simulink model "complete_model_sim"  (R2023b)
settings: Solver=VariableStepAuto  StartTime=0.0  StopTime=5e3  RelTol=1e-3
values from neighbouring files (symbols this model uses):
  a = 6.851221970532768e+03    (= 6851.22197053)    [complete_model.m]
  alpha1 = 0.05    [complete_model.m]
  alpha2 = 0.15    [complete_model.m]
  alpha3 = 0.8    [complete_model.m]
  D = squeeze(out.D)    [complete_model.m]
  e = 0.001830122216180    (= 0.00183012221618)    [complete_model.m]
  FOV_earth = deg2rad(33)    [complete_model.m]
  freq_earth = 30    [complete_model.m]
  freq_mag = 30    [complete_model.m]
  freq_sun = 30    [complete_model.m]
  H0 = sqrt(g01^2+g11^2+h11^2)*1e-9    [complete_model.m]
  I = I + (y(i + 1) + y(i) ) * (t(i + 1) - t(i)) * 0.5    [compute_integral.m]
  incl = deg2rad(11.5)    [complete_model.m]
  jb = [0.01; 0.05; 0.01]    [complete_model.m]
  k_gain = (4*pi/T) * (1 + sin(chsi)) * I1_retr    [complete_model.m]
  mu = astroConstants(13)    [complete_model.m]
  n = sqrt(mu/a^3)    [complete_model.m]
  omega0 = -0.06 + 0.12 * rand(3,1)    [complete_model.m]
  omegaE = deg2rad(15)/3600    [complete_model.m]
  rs = -rr    [complete_model.m]
  Rt = astroConstants(23)    [complete_model.m]
  s0 = 2*pi*rand(3,1)    [complete_model.m]
  tol = 0.2    [complete_model.m]
undefined symbols (not defined in the file or in its folder): FOV_sun, Iinv, magnitude
libraries: simulink x16, vrlib x13, matrix_library x12, cstblocks x6, dspsolvers x4, sharedutil x2, aerolibutil x2, dspfactors x1, dspmathops x1
(part 1 of 2)
settings Model: Creator=marcellopareschi  LastModifiedBy=turcu

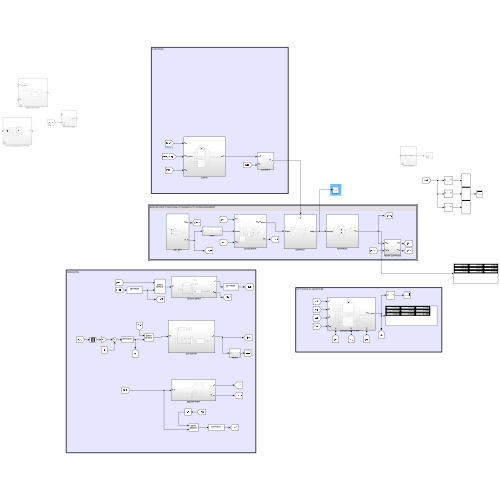
[thumbnail: Simulink's stored preview of the top-level diagram]
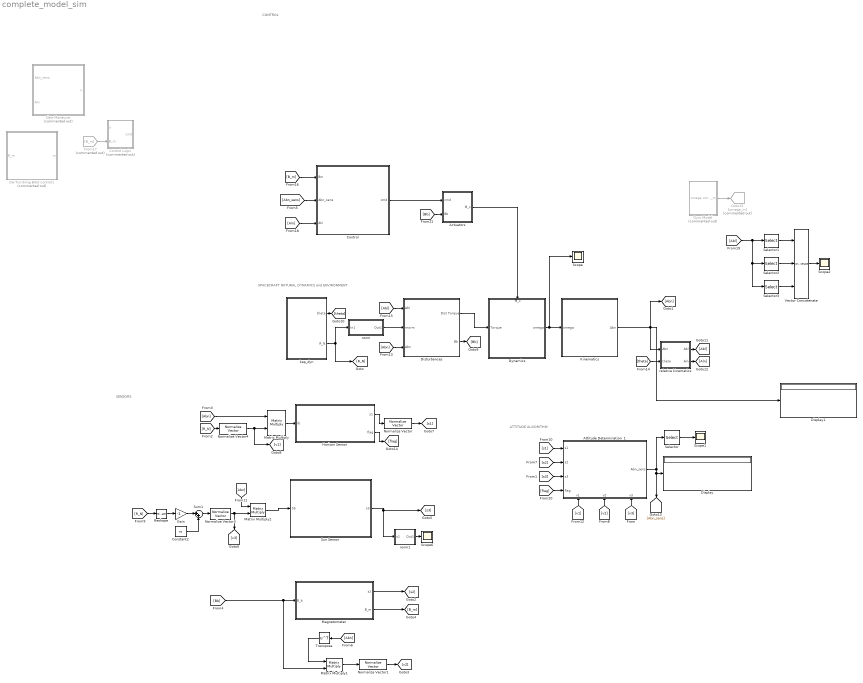
== system complete_model_sim ==
  note: SPACECRAFT NATURAL DYNAMICS and ENVIRONMENT
  note: CONTROL
  note: ATTITUDE ALGORITHM
  note: SENSORS
  " Actuators" : Subsystem
  Attitude Determination  1 : Subsystem
      settings: PortSchema="{\"entries\":[{\"content\":{\"sides\":[{\"content\":{\"connectorIds\":[\"In1\",\"In2\",\"In3\",\"In4\"]},\"type\":\"ConnectorPlacement.EquallySpacedRectSide\",\"uuid\":\"730966cf-d0d7-44a0-92f0-b5324480e7cc\"},{\"content\":{\"connectorIds\":[\"Out1\"],\"side\":\"RIGHT\"},\"type\":\"ConnectorPlacement.EquallySpacedRectSide\",\"uuid\":\"c83e6b57-46fe-4a45-9824-d3495e15bf6a\"},{\"content\":{\"side\":\"TOP\"},\"type\":\"ConnectorPlacement.EquallySpacedRectSide\",\"uuid\":\"4938c298-c2b3-45b7-bcb0-70b8132dabc6\"},{\"content\":{\"connectorIds\":[\"In5\",\"In6\",\"In7\"],\"side\":\"BOTTOM\"},\"type\":\"ConnectorPlacement.EquallySpacedRectSide\",\"uuid\":\"6d6a244e-80db-423b-a0a5-9a5face48fcb\"}]},\"type\":\"ConnectorPlacement.EquallySpacedConnector\",\"uuid\":\"7eb6767d-3ff0-4577-86c9-ebc5e763f220\"}],\"packageUris\":[\"http://schema.mathworks.com/mf0/Connector/R2020b\"],\"version\":\"1.0\"}"
  Constant2 : Constant  Value=rs
  Control : Subsystem
  Control Logic : Subsystem  Commented=on
  De-Tumbling Bdot control1 : Subsystem  Commented=on
  Display : Display
  Display1 : Display
  Disturbances : Subsystem
  Dynamics : Subsystem
      settings: PortSchema="{\"entries\":[{\"content\":{\"sides\":[{\"content\":{\"connectorIds\":[\"In1\"]},\"type\":\"ConnectorPlacement.EquallySpacedRectSide\",\"uuid\":\"c50eaaef-bc5a-4b30-975a-dad3b72c53e1\"},{\"content\":{\"connectorIds\":[\"Out1\"],\"side\":\"RIGHT\"},\"type\":\"ConnectorPlacement.EquallySpacedRectSide\",\"uuid\":\"08d23e91-5daf-4f03-95f9-71d6696597c3\"},{\"content\":{\"connectorIds\":[\"In2\"],\"side\":\"TOP\"},\"type\":\"ConnectorPlacement.EquallySpacedRectSide\",\"uuid\":\"7ec65280-cc3e-44b1-8843-81c3a216d755\"}]},\"type\":\"ConnectorPlacement.EquallySpacedConnector\",\"uuid\":\"721d018a-ab6c-4a15-8dbf-409a72b03ba1\"}],\"packageUris\":[\"http://schema.mathworks.com/mf0/Connector/R2020b\"],\"version\":\"1.0\"}"
  From17 : From  Commented=on  GotoTag=B_m
  Gain : Gain  Gain=-1
  Goto15 : Goto  Commented=on  GotoTag=omega_m
  Gyro Model : Subsystem  Commented=on
  Horizon Sensor : Subsystem
  Kinematics : Subsystem
  Magnetometer : Subsystem
  Matrix Multiply : Product  Multiplication=Matrix(*)
  Matrix Multiply1 : Product  Multiplication=Matrix(*)
  Matrix Multiply2 : Product  Multiplication=Matrix(*)
  Normalize Vector{,1,3..4} (4 alike) : vrlib/Utilities/Normalize Vector  maxzero=0
  Reshape : Reshape  OutputDimensionality=Column vector (2-D)
  Scope{,1..2,6} (4 alike) : Scope
  Selector : Selector  NumberOfDimensions=2  InputPortWidth=3  IndexOptions=Index vector (dialog),Index vector (dialog)  Indices=1,1  OutputSizes=1,1
  Selector1 : Selector  NumberOfDimensions=2  InputPortWidth=3  IndexOptions=Index vector (dialog),Index vector (dialog)  Indices=3,2  OutputSizes=1,1
  Selector2 : Selector  NumberOfDimensions=2  InputPortWidth=3  IndexOptions=Index vector (dialog),Index vector (dialog)  Indices=1,3  OutputSizes=1,1
  Selector3 : Selector  NumberOfDimensions=2  InputPortWidth=3  IndexOptions=Index vector (dialog),Index vector (dialog)  Indices=2,1  OutputSizes=1,1
  Slew Maneuver : Subsystem  Commented=on
  Sum1 : Sum  Inputs=|++
  Sun Sensor : Subsystem
  Transpose : Math  Operator=transpose
  Vector Concatenate : Concatenate  NumInputs=3
  kep_dyn : Subsystem
  norm : Subsystem
  norm1 : Subsystem
  relative kinematics : Subsystem
  wires:
  Normalize Vector3/1 -> Matrix Multiply2/2, [v3]
  Magnetometer/1(s2) -> [s2]
  Disturbances/2(Bb) -> [Bb]
  [Abn] -> Transpose/1
  Matrix Multiply1/1 -> Normalize Vector1/1
  Transpose/1 -> Matrix Multiply1/1
  [theta] -> relative kinematics/2(theta)
  [v1] -> Attitude Determination  1/5(v1)
  [Abn] -> Matrix Multiply/1
  [R_N] -> Reshape/1
  Gain/1 -> Sum1/1
  [Bb] -> Matrix Multiply1/2, Magnetometer/1(B_b)
  Normalize Vector4/1 -> [v1], Matrix Multiply/2
  [s3] -> Attitude Determination  1/3(s3)
  Normalize Vector1/1 -> [v2]
  " Actuators"/1(M_c) -> Dynamics/2(M_c)
  Magnetometer/2("B_m ") -> [B_m]
  Sun Sensor/1(s3) -> norm1/1(s1), [s3]
  [R_N] -> Normalize Vector4/1
  Constant2/1 -> Sum1/2
  kep_dyn/1(theta) -> [theta]
  [s2] -> Attitude Determination  1/2(s2)
  Matrix Multiply/1 -> Horizon Sensor/1(rb)
  Reshape/1 -> Gain/1
  [Abl] -> Disturbances/1(Abl)
  Normalize Vector/1 -> [s1]
  [v3] -> Attitude Determination  1/7(v3)
  [s1] -> Attitude Determination  1/1(s1)
  kep_dyn/2(R_N) -> [R_N], norm/1(In1)
  Sum1/1 -> Normalize Vector3/1
  Attitude Determination  1/1(Abn_sens) -> [Abn_sens], Display/1, Selector/1
  relative kinematics/1(Abl) -> [Abl]
  Kinematics/1(Abn) -> [Abn], Display1/1, relative kinematics/1(Abn)
  relative kinematics/2(Aln) -> [Aln]
  Selector/1 -> Scope1/1
  [Abn] -> Disturbances/3(Abn)
  norm/1(Out1) -> Disturbances/2(rnorm)
  [Abn] -> Matrix Multiply2/1
  Disturbances/1(Dist Torque) -> Dynamics/1(Torque)
  Dynamics/1(omega) -> Scope/1, Kinematics/1(omega)
  [v2] -> Attitude Determination  1/6(v2)
  Horizon Sensor/1(s1) -> Normalize Vector/1
  Matrix Multiply2/1 -> Sun Sensor/1(Sb)
  norm1/1(Out1) -> Scope6/1
  Gyro Model/1(omega_m) -> Goto15/1
  [Bb] -> " Actuators"/2(Bb)
  From17/1 -> Control Logic/2(B_m)
  [B_m] -> Control/1(Bm)
  [Abn_sens] -> Control/2(Abn_sens)
  [Aln] -> Control/3(Aln)
  Control/1(cmd) -> " Actuators"/1(cmd)
  [Abl] -> Selector3/1, Selector2/1, Selector1/1
  Selector2/1 -> Vector Concatenate/2
  Selector3/1 -> Vector Concatenate/3
  Selector1/1 -> Vector Concatenate/1
  Vector Concatenate/1 -> Scope2/1
  Horizon Sensor/2(flag) -> [flag]
  [flag] -> Attitude Determination  1/4(flag)

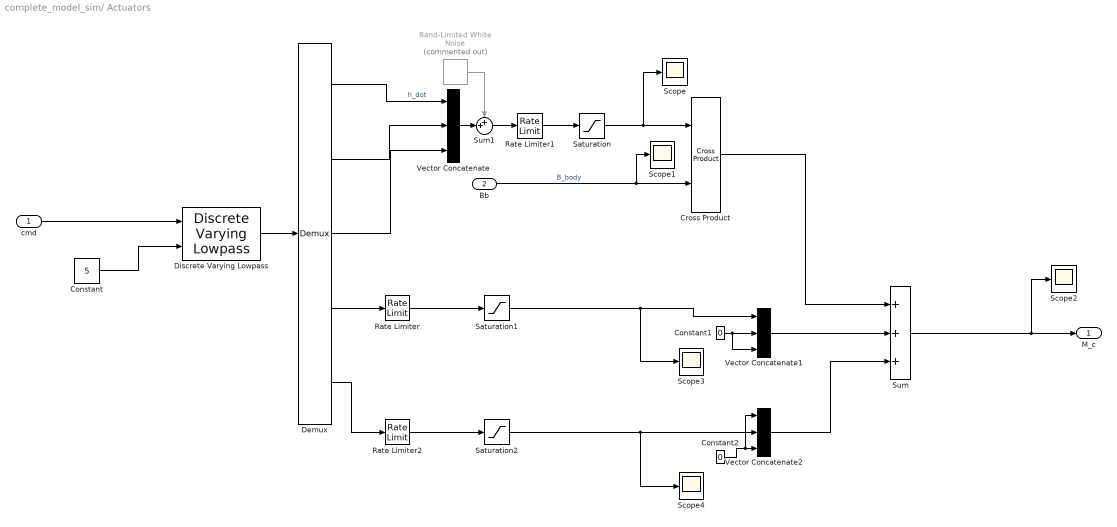
== system complete_model_sim/ Actuators ==
  cmd : Inport
  Bb : Inport  Port=2
  Band-Limited White Noise : simulink/Sources/Band-Limited White Noise  Commented=on  Cov=[0.1]  Ts=1/30  seed=[23341]
  Constant : Constant  Value=5
  Constant1 : Constant  Value=0
  Constant2 : Constant  Value=0
  Cross Product : matrix_library/Cross Product
  Demux : Demux  Outputs=5
  Discrete Varying Lowpass : cstblocks/Linear Parameter Varying/Discrete Varying Lowpass  N=2  w0=0  Ts=1/30
  Rate Limiter : RateLimiter
  Rate Limiter1 : RateLimiter  RisingSlewLimit=10  FallingSlewLimit=-10
  Rate Limiter2 : RateLimiter
  Saturation : Saturate  UpperLimit=150  LowerLimit=-150
  Saturation1 : Saturate
  Saturation2 : Saturate
  Scope{,1..4} (5 alike) : Scope
  Sum : Sum  Inputs=+++
  Sum1 : Sum  Inputs=++|
  Vector Concatenate : Concatenate  NumInputs=3
  Vector Concatenate1 : Concatenate  NumInputs=3
  Vector Concatenate2 : Concatenate  NumInputs=3
  M_c : Outport
  wires:
  Bb/1 -> Scope1/1, Cross Product/2  "B_body"
  Rate Limiter1/1 -> Saturation/1
  Band-Limited White Noise/1 -> Sum1/1
  Sum1/1 -> Rate Limiter1/1
  Saturation/1 -> Scope/1, Cross Product/1
  Vector Concatenate/1 -> Sum1/2
  Constant1/1 -> Vector Concatenate1/3, Vector Concatenate1/2
  Sum/1 -> Scope2/1, M_c/1
  Rate Limiter/1 -> Saturation1/1
  Saturation1/1 -> Scope3/1, Vector Concatenate1/1
  Demux/1 -> Vector Concatenate/1  "h_dot"
  Demux/2 -> Vector Concatenate/2
  Demux/3 -> Vector Concatenate/3
  Demux/4 -> Rate Limiter/1
  Saturation2/1 -> Vector Concatenate2/2, Scope4/1
  Constant2/1 -> Vector Concatenate2/1, Vector Concatenate2/3
  Rate Limiter2/1 -> Saturation2/1
  Demux/5 -> Rate Limiter2/1
  Vector Concatenate1/1 -> Sum/2
  Cross Product/1 -> Sum/1
  Vector Concatenate2/1 -> Sum/3
  Constant/1 -> Discrete Varying Lowpass/2
  Discrete Varying Lowpass/1 -> Demux/1
  cmd/1 -> Discrete Varying Lowpass/1

== system complete_model_sim/Attitude Determination  1 ==
  s1 : Inport
  s2 : Inport  Port=2
  s3 : Inport  Port=3
  flag : Inport  Port=4
  v1 : Inport  Port=5
  v2 : Inport  Port=6
  v3 : Inport  Port=7
  Enabled Subsystem : Subsystem  TreatAsAtomicUnit=on
  Merge : Merge
  NOT : Logic  Operator=NOT  IconShape=distinctive  AllPortsSameDT=off  OutDataTypeStr=boolean
  Statistical Method : Subsystem  TreatAsAtomicUnit=on
  Abn_sens : Outport
  wires:
  flag/1 -> NOT/1, Statistical Method/Enable
  s1/1 -> Statistical Method/1(s1)
  s2/1 -> Enabled Subsystem/1(q), Statistical Method/2(s2)
  s3/1 -> Enabled Subsystem/2(p), Statistical Method/3(s3)
  v1/1 -> Statistical Method/4(v1)
  v2/1 -> Enabled Subsystem/3(b), Statistical Method/5(v2)
  v3/1 -> Enabled Subsystem/4(a), Statistical Method/6(v3)
  NOT/1 -> Enabled Subsystem/Enable
  Statistical Method/1(Abn_sens) -> Merge/1
  Enabled Subsystem/1(A_bn_sens) -> Merge/2
  Merge/1 -> Abn_sens/1

== system complete_model_sim/Control ==
  Bm : Inport
  Abn_sens : Inport  Port=2
  Aln : Inport  Port=3
  De-Tumbling Bdot control1 : Subsystem
  Merge : Merge
  NOT : Logic  Operator=NOT  IconShape=distinctive  AllPortsSameDT=off  OutDataTypeStr=boolean
  Scope1 : Scope
  Slew Maneuver : Subsystem
  Unit Delay : UnitDelay  InitialCondition=1  SampleTime=-1  HasFrameUpgradeWarning=on
  cmd : Outport
  wires:
  Unit Delay/1 -> NOT/1, Scope1/1, De-Tumbling Bdot control1/Enable
  De-Tumbling Bdot control1/2(flag) -> Unit Delay/1
  Bm/1 -> Slew Maneuver/3(B_m), De-Tumbling Bdot control1/1(B_m)
  Abn_sens/1 -> Slew Maneuver/1(Abn_sens)
  Aln/1 -> Slew Maneuver/2(Aln)
  NOT/1 -> Slew Maneuver/Enable
  Slew Maneuver/1(cmd) -> Merge/2
  De-Tumbling Bdot control1/1(cmd) -> Merge/1
  Merge/1 -> cmd/1

== system complete_model_sim/Control Logic ==
  u : Inport
  B_m : Inport  Port=2
  Abs1 : Abs  SaturateOnIntegerOverflow=off
  Compare To Constant : simulink/Logic and Bit Operations/Compare To Constant  relop=>  const=1e-5  OutDataTypeStr=boolean
  Discrete Derivative : simulink/Discrete/Discrete Derivative  gainval=1.0  ICPrevScaledInput=0.0  OutMin=[]  OutMax=[]  OutDataType=fixdt(1, 16)  OutScaling=2^-10  DoSatur=off
  Merge1 : Merge
  NOT : Logic  Operator=NOT  IconShape=distinctive  AllPortsSameDT=off  OutDataTypeStr=boolean
  Scope : Scope
  Selector1 : Selector  InputPortWidth=3  IndexOptions=Index vector (dialog)  Indices=1  OutputSizes=1
  Subsystem : Subsystem
  Subsystem1 : Subsystem
  norm : Subsystem
  cmd : Outport
  wires:
  Abs1/1 -> Compare To Constant/1
  Selector1/1 -> Abs1/1
  NOT/1 -> Subsystem/Enable
  Subsystem1/1(Out1) -> Merge1/1
  Compare To Constant/1 -> NOT/1, Subsystem1/Enable
  Subsystem/1(Out1) -> Merge1/2
  B_m/1 -> Discrete Derivative/1, Selector1/1, Subsystem/1(Bm), Subsystem1/1(B_m)
  u/1 -> Subsystem/2(u), Subsystem1/2(u)
  Merge1/1 -> cmd/1
  Discrete Derivative/1 -> norm/1(In1)
  norm/1(Out1) -> Scope/1

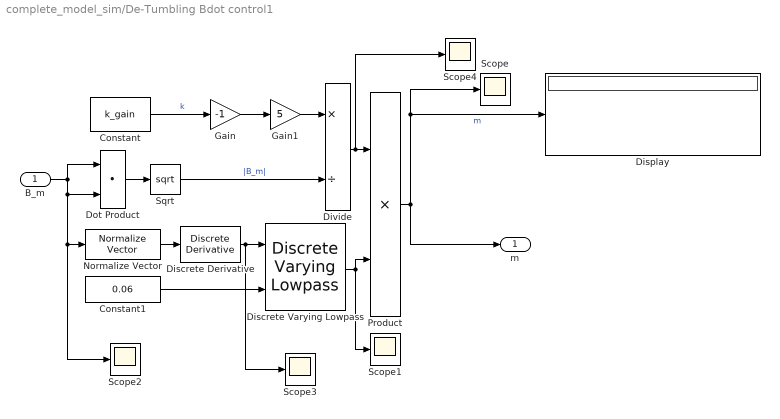
== system complete_model_sim/De-Tumbling Bdot control1 ==
  B_m : Inport
  Constant : Constant  Value=k_gain
  Constant1 : Constant  Value=0.06  SampleTime=1/30
  Discrete Derivative : simulink/Discrete/Discrete Derivative  gainval=1.0  ICPrevScaledInput=0.0  OutMin=[]  OutMax=[]  OutDataType=fixdt(1, 16)  OutScaling=2^-10  DoSatur=off
  Discrete Varying Lowpass : cstblocks/Linear Parameter Varying/Discrete Varying Lowpass  N=1  w0=0  Ts=1/30
  Display : Display
  Divide : Product  Inputs=*/
  Dot Product : DotProduct  OutDataTypeStr=Inherit: Inherit via internal rule
  Gain : Gain  Gain=-1
  Gain1 : Gain  Gain=5
  Normalize Vector : vrlib/Utilities/Normalize Vector  maxzero=0
  Product : Product
  Scope{,1..4} (5 alike) : Scope
  Sqrt : Sqrt
  m : Outport
  wires:
  Dot Product/1 -> Sqrt/1
  Constant/1 -> Gain/1  "k"
  Gain/1 -> Gain1/1
  Divide/1 -> Scope4/1, Product/1
  Product/1 -> m/1, Scope/1, Display/1  "m"
  Sqrt/1 -> Divide/2  "|B_m|"
  Gain1/1 -> Divide/1
  Normalize Vector/1 -> Discrete Derivative/1
  B_m/1 -> Dot Product/2, Scope2/1, Normalize Vector/1, Dot Product/1
  Discrete Derivative/1 -> Scope3/1, Discrete Varying Lowpass/1
  Discrete Varying Lowpass/1 -> Scope1/1, Product/2
  Constant1/1 -> Discrete Varying Lowpass/2

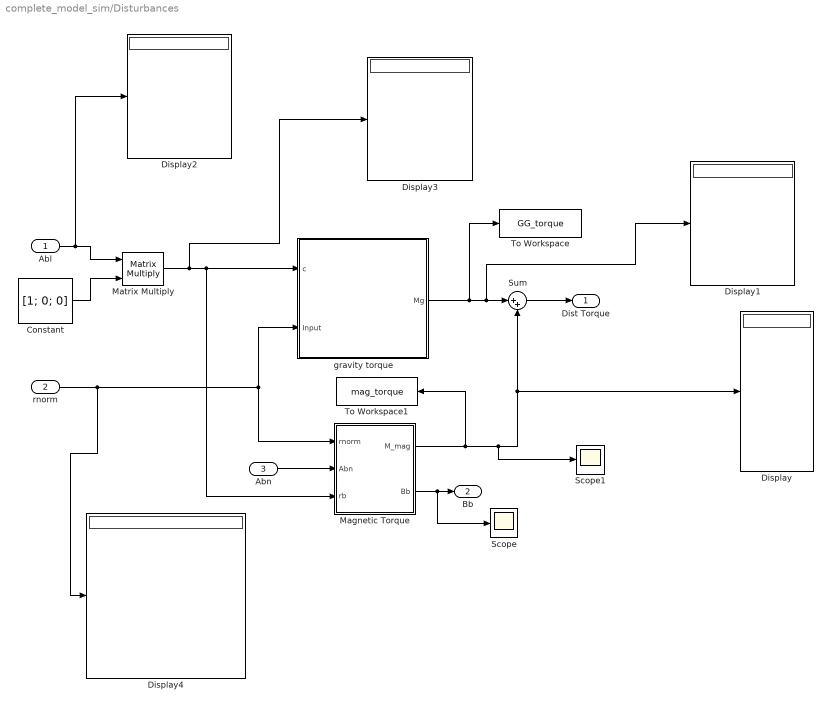
== system complete_model_sim/Disturbances ==
  Abl : Inport
  rnorm : Inport  Port=2
  Abn : Inport  Port=3
  Constant : Constant  Value=[1; 0; 0]
  Display{,1..4} (5 alike) : Display
  "Magnetic Torque " : Subsystem
  Matrix Multiply : Product  Multiplication=Matrix(*)
  Scope : Scope
  Scope1 : Scope
  Sum : Sum  Inputs=|++
  To Workspace : ToWorkspace  VariableName=GG_torque  SampleTime=-1
  To Workspace1 : ToWorkspace  VariableName=mag_torque  SampleTime=-1
  gravity torque : Subsystem
  Dist Torque : Outport
  Bb : Outport  Port=2
  wires:
  Abl/1 -> Display2/1, Matrix Multiply/1
  Constant/1 -> Matrix Multiply/2
  Matrix Multiply/1 -> Display3/1, "Magnetic Torque "/3(rb), gravity torque/1(c)
  rnorm/1 -> Display4/1, "Magnetic Torque "/1(rnorm), gravity torque/2(Input)
  Abn/1 -> "Magnetic Torque "/2(Abn)
  gravity torque/1(Mg) -> To Workspace/1, Display1/1, Sum/1
  "Magnetic Torque "/1(M_mag) -> To Workspace1/1, Scope1/1, Sum/2, Display/1
  Sum/1 -> Dist Torque/1
  "Magnetic Torque "/2(Bb) -> Scope/1, Bb/1

== system complete_model_sim/Dynamics ==
  Torque : Inport
  M_c : Inport  Port=2
  Constant : Constant  Value=I
  Constant1 : Constant  Value=Iinv
  Cross Product : matrix_library/Cross Product
  Integrator : Integrator  InitialCondition=omega0
  Product : Product  Multiplication=Matrix(*)
  Product1 : Product  Multiplication=Matrix(*)
  Scope : Scope
  Scope1 : Scope
  Sum : Sum  Inputs=+++
  To Workspace : ToWorkspace  VariableName=omegab  SampleTime=-1
  omega : Outport
  wires:
  Constant/1 -> Product/1
  Product1/1 -> Integrator/1
  Integrator/1 -> Product/2, Cross Product/2, Scope/1, To Workspace/1, omega/1
  Product/1 -> Cross Product/1
  Constant1/1 -> Product1/1
  Cross Product/1 -> Sum/2
  Sum/1 -> Product1/2
  Torque/1 -> Sum/3
  M_c/1 -> Scope1/1, Sum/1

== system complete_model_sim/Gyro Model ==
  omega : Inport
  Constant : Constant
  Discrete Varying Lowpass : cstblocks/Linear Parameter Varying/Discrete Varying Lowpass  N=2  w0=0  Ts=1
  Integrator : Integrator
  Random Number : RandomNumber  Variance=(9.6963*1e-7)^2  SampleTime=0.1
  Random Number1 : RandomNumber  Variance=(9.6963*1e-7)^2  SampleTime=0.1
  Random Number2 : RandomNumber  Variance=(9.6963*1e-7)^2  SampleTime=0.1
  Random Number3 : RandomNumber  Variance=(2.3522*1e-5)^2  SampleTime=0.1
  Random Number4 : RandomNumber  Variance=(2.3522*1e-5)^2  SampleTime=0.1
  Random Number5 : RandomNumber  Variance=(2.3522*1e-5)^2  SampleTime=0.1
  Sum : Sum  Inputs=+++
  Vector Concatenate : Concatenate  NumInputs=3
  Vector Concatenate1 : Concatenate  NumInputs=3
  omega_m : Outport
  wires:
  Random Number1/1 -> Vector Concatenate/2
  Random Number/1 -> Vector Concatenate/1
  Random Number2/1 -> Vector Concatenate/3
  Vector Concatenate/1 -> Integrator/1
  Random Number3/1 -> Vector Concatenate1/1
  Random Number4/1 -> Vector Concatenate1/2
  Random Number5/1 -> Vector Concatenate1/3
  omega/1 -> Sum/2
  Vector Concatenate1/1 -> Sum/1
  Integrator/1 -> Sum/3
  Sum/1 -> Discrete Varying Lowpass/1
  Discrete Varying Lowpass/1 -> omega_m/1
  Constant/1 -> Discrete Varying Lowpass/2

== system complete_model_sim/Horizon Sensor ==
  rb : Inport
  EH sensor modeling : Subsystem
  FOV CHECK : Subsystem
  Product1 : Product
  Scope : Scope
  s1 : Outport
  flag : Outport  Port=2
  wires:
  rb/1 -> FOV CHECK/1(rb), Product1/2
  Product1/1 -> EH sensor modeling/1(rb)
  EH sensor modeling/1(q) -> s1/1  "direction of earth"
  FOV CHECK/1(b) -> Product1/1, Scope/1, flag/1

== system complete_model_sim/Kinematics ==
  omega : Inport
  Kinematics 312 : Subsystem
  Kinematics 313 : Subsystem
  Merge : Merge
  NOT : Logic  Operator=NOT  IconShape=distinctive  AllPortsSameDT=off  OutDataTypeStr=boolean
  System switcher : Subsystem
  To Workspace : ToWorkspace  VariableName=A  SaveFormat=Timeseries  SampleTime=-1
  Abn : Outport
  wires:
  NOT/1 -> Kinematics 313/Enable
  omega/1 -> Kinematics 312/1(w), Kinematics 313/1(w)
  System switcher/1(flag) -> Kinematics 312/Enable, NOT/1
  Kinematics 313/1(A) -> Merge/2
  Merge/1 -> Abn/1, To Workspace/1  "A"
  Kinematics 312/1(A) -> Merge/1

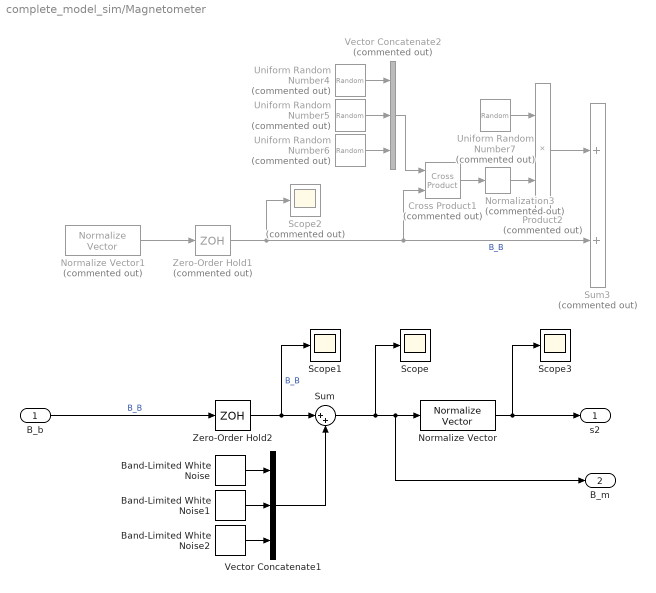
== system complete_model_sim/Magnetometer ==
  B_b : Inport
  Band-Limited White Noise : simulink/Sources/Band-Limited White Noise  Cov=[1.18^2 *1e-18]  Ts=1/30  seed=[23341]
  Band-Limited White Noise1 : simulink/Sources/Band-Limited White Noise  Cov=[1.18^2 *1e-18]  Ts=1/30  seed=[23341]
  Band-Limited White Noise2 : simulink/Sources/Band-Limited White Noise  Cov=[1.18^2 *1e-18]  Ts=1/30  seed=[23341]
  Cross Product1 : matrix_library/Cross Product  Commented=on
  Normalization3 : dspmathops/Normalization  Commented=on  NormType=2-norm  Bias=1e-10  NormOver=Each column  Dimension=1  roundingMode=Floor  overflowMode=off  accumDataTypeStr=Inherit: Same as product output  accumLastDataTypeStr=Inherit: Same as product output  outputDataTypeStr=Inherit: Same as product output  outputMin=[]  outputMax=[]  outputLastDataTypeStr=Inherit: Same as product output
  Normalize Vector : vrlib/Utilities/Normalize Vector  maxzero=0
  Normalize Vector1 : vrlib/Utilities/Normalize Vector  Commented=on  maxzero=0
  Product2 : Product  Commented=on
  Scope : Scope
  Scope1 : Scope
  Scope2 : Scope  Commented=on
  Scope3 : Scope
  Sum : Sum  Inputs=|++
  Sum3 : Sum  Commented=on
  Uniform Random Number4 : UniformRandomNumber  Commented=on  SampleTime=1/30
  Uniform Random Number5 : UniformRandomNumber  Commented=on  SampleTime=1/30
  Uniform Random Number6 : UniformRandomNumber  Commented=on  SampleTime=1/30
  Uniform Random Number7 : UniformRandomNumber  Commented=on  Minimum=0  Maximum=tan(deg2rad(0.5))*0.1  SampleTime=1/30
  Vector Concatenate1 : Concatenate  NumInputs=3
  Vector Concatenate2 : Concatenate  Commented=on  NumInputs=3
  Zero-Order Hold1 : ZeroOrderHold  Commented=on  SampleTime=1/30
  Zero-Order Hold2 : ZeroOrderHold  SampleTime=1/freq_mag
  s2 : Outport
  "B_m " : Outport  Port=2
  wires:
  Zero-Order Hold1/1 -> Cross Product1/2, Sum3/2, Scope2/1  "B_B"
  Product2/1 -> Sum3/1
  Normalization3/1 -> Product2/2
  Uniform Random Number4/1 -> Vector Concatenate2/1
  Uniform Random Number6/1 -> Vector Concatenate2/3
  Vector Concatenate2/1 -> Cross Product1/1
  Cross Product1/1 -> Normalization3/1
  Uniform Random Number5/1 -> Vector Concatenate2/2
  Uniform Random Number7/1 -> Product2/1
  Zero-Order Hold2/1 -> Scope1/1, Sum/1  "B_B"
  Band-Limited White Noise2/1 -> Vector Concatenate1/3
  Band-Limited White Noise1/1 -> Vector Concatenate1/2
  Band-Limited White Noise/1 -> Vector Concatenate1/1
  Normalize Vector/1 -> s2/1, Scope3/1
  Vector Concatenate1/1 -> Sum/2
  Sum/1 -> Scope/1, "B_m "/1, Normalize Vector/1
  Normalize Vector1/1 -> Zero-Order Hold1/1
  B_b/1 -> Zero-Order Hold2/1  "B_B"

== system complete_model_sim/Slew Maneuver ==
  Abn_sens : Inport
  Aln : Inport  Port=2
  Gain : Gain  Gain=-1
  Gain2 : Gain  Gain=-0.01
  Matrix Multiply : Product  Multiplication=Matrix(*)
  Scope : Scope
  Sum : Sum
  Transpose : Math  Operator=transpose
  compute alphadots : Subsystem
  compute alphas : Subsystem
  u : Outport
  wires:
  Aln/1 -> Transpose/1
  Transpose/1 -> Matrix Multiply/2
  Abn_sens/1 -> Matrix Multiply/1, compute alphadots/1(Abn)
  Matrix Multiply/1 -> compute alphas/1(Abl), compute alphadots/2(Abl)
  compute alphadots/1(Alphadots) -> Gain/1
  compute alphas/1(estimated state) -> Scope/1, Gain2/1
  Gain/1 -> Sum/1
  Gain2/1 -> Sum/2
  Sum/1 -> u/1

== system complete_model_sim/Sun Sensor ==
  Sb : Inport
  Constant : Constant
  FOV CHECK : Subsystem
  Product : Product
  Scope : Scope
  Sun Sensor Modeling : Subsystem
  s3 : Outport
  wires:
  Sb/1 -> Product/2, FOV CHECK/1(In1)  "Sb"
  Sun Sensor Modeling/1(s3) -> s3/1
  Product/1 -> Sun Sensor Modeling/1(Sb)  "Sb"
  Constant/1 -> Product/1
  FOV CHECK/1(b) -> Scope/1

== system complete_model_sim/kep_dyn ==
  A_np : Constant  Value=A_pn'
  Constant : Constant  Value=0
  Constant1 : Constant  Value=e
  Cos : Trigonometry  Operator=cos
  Integrator : Integrator
  Matrix Multiply : Product  Multiplication=Matrix(*)
  Product2 : Product
  Sin : Trigonometry
  Vector Concatenate : Concatenate  NumInputs=3
  r_norm : Subsystem
  theta integration : Subsystem
      settings: PortSchema="{\"entries\":[{\"content\":{\"sides\":[{\"content\":{\"connectorIds\":[\"In1\"]},\"type\":\"ConnectorPlacement.EquallySpacedRectSide\",\"uuid\":\"3f1b1ec9-07ed-4eb1-9e41-630dc5613e97\"},{\"content\":{\"connectorIds\":[\"Out1\",\"In2\"],\"side\":\"RIGHT\"},\"type\":\"ConnectorPlacement.EquallySpacedRectSide\",\"uuid\":\"22d0f7bc-714c-4365-a26c-07047ff4be14\"},{\"content\":{\"side\":\"TOP\"},\"type\":\"ConnectorPlacement.EquallySpacedRectSide\",\"uuid\":\"875f7006-d698-4730-93ae-1a7d05f24054\"}]},\"type\":\"ConnectorPlacement.EquallySpacedConnector\",\"uuid\":\"799b65b1-faea-432b-9f3f-2d21984184cd\"}],\"packageUris\":[\"http://schema.mathworks.com/mf0/Connector/R2020b\"],\"version\":\"1.0\"}"
  theta : Outport
  R_N : Outport  Port=2
  wires:
  Integrator/1 -> Sin/1, Cos/1, r_norm/2(theta), theta/1, theta integration/1(theta)
  theta integration/1(theta_dot) -> Integrator/1
  Constant/1 -> Vector Concatenate/3
  Cos/1 -> Vector Concatenate/1
  Constant1/1 -> r_norm/1(e), theta integration/2(e)
  r_norm/1(r) -> Product2/1
  Vector Concatenate/1 -> Product2/2
  Sin/1 -> Vector Concatenate/2
  A_np/1 -> Matrix Multiply/1
  Product2/1 -> Matrix Multiply/2
  Matrix Multiply/1 -> R_N/1

== system complete_model_sim/norm ==
  In1 : Inport
  Dot Product : DotProduct  OutDataTypeStr=Inherit: Inherit via internal rule
  Sqrt : Sqrt
  Out1 : Outport
  wires:
  In1/1 -> Dot Product/1, Dot Product/2
  Dot Product/1 -> Sqrt/1
  Sqrt/1 -> Out1/1

== system complete_model_sim/norm1 ==
  s1 : Inport
  Dot Product : DotProduct  OutDataTypeStr=Inherit: Inherit via internal rule
  Square Root : Sqrt
  Out1 : Outport
  wires:
  s1/1 -> Dot Product/1, Dot Product/2
  Dot Product/1 -> Square Root/1
  Square Root/1 -> Out1/1

== system complete_model_sim/relative kinematics ==
  Abn : Inport
  theta : Inport  Port=2
  Constant : Constant  Value=A_pn'
  Matrix Multiply : Product  Multiplication=Matrix(*)
  Matrix Multiply2 : Product  Multiplication=Matrix(*)
  Subsystem : Subsystem
  Transpose : Math  Operator=transpose
  Abl : Outport
  Aln : Outport  Port=2
  wires:
  Abn/1 -> Matrix Multiply2/1
  Matrix Multiply/1 -> Transpose/1, Matrix Multiply2/2  "A_nl"
  Matrix Multiply2/1 -> Abl/1
  theta/1 -> Subsystem/1(theta)
  Subsystem/1(A_PL) -> Matrix Multiply/2  "A_PL"
  Constant/1 -> Matrix Multiply/1  "A_np"
  Transpose/1 -> Aln/1

== system complete_model_sim/Attitude Determination  1/Enabled Subsystem ==
  q : Inport
  p : Inport  Port=2
  b : Inport  Port=3
  a : Inport  Port=4
  Enable : EnablePort
  Matrix Multiply : Product  Multiplication=Matrix(*)
  S : Subsystem
  Transpose : Math  Operator=transpose
  V : Subsystem
  A_bn_sens : Outport
  wires:
  V/1(V) -> Transpose/1
  S/1(S) -> Matrix Multiply/1
  Transpose/1 -> Matrix Multiply/2
  Matrix Multiply/1 -> A_bn_sens/1
  q/1 -> S/1(q)
  p/1 -> S/2(p)
  b/1 -> V/1(b)
  a/1 -> V/2(a)

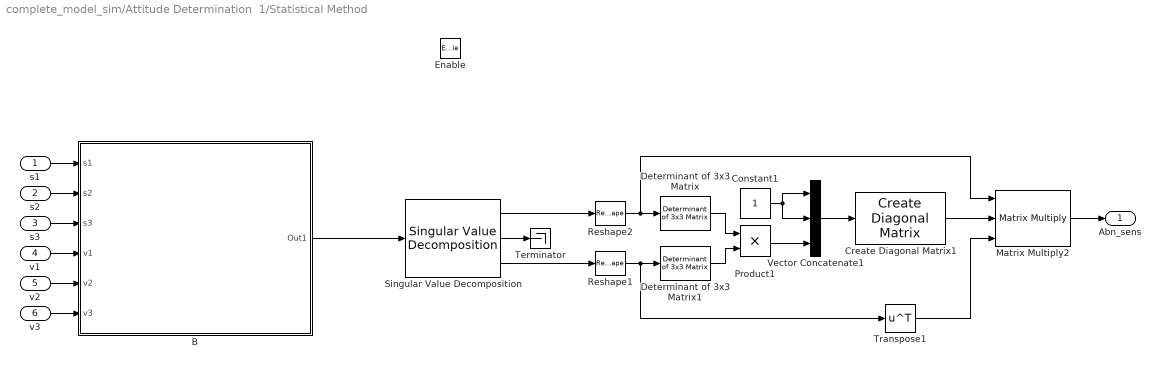
== system complete_model_sim/Attitude Determination  1/Statistical Method ==
  s1 : Inport
  s2 : Inport  Port=2
  s3 : Inport  Port=3
  v1 : Inport  Port=4
  v2 : Inport  Port=5
  v3 : Inport  Port=6
  Enable : EnablePort
  B : Subsystem
  Constant1 : Constant
  Create Diagonal Matrix1 : matrix_library/Create Diagonal Matrix
      settings: LibrarySourceBlock=|
      | simulink/Matrix
      | Operations/Create Diagonal
      | Matrix
  Determinant of 3x3 Matrix : sharedutil/Determinant of 3x3 Matrix  aMode=aMode
      settings: LibrarySourceBlock=|
      | aerolibutil/Determinant of
      | 3x3 Matrix
  Determinant of 3x3 Matrix1 : sharedutil/Determinant of 3x3 Matrix  aMode=aMode
      settings: LibrarySourceBlock=|
      | aerolibutil/Determinant of
      | 3x3 Matrix
  Matrix Multiply2 : Product  Inputs=3  Multiplication=Matrix(*)
  Product1 : Product
  Reshape1 : Reshape  OutputDimensionality=Customize  OutputDimensions=[3,3]
  Reshape2 : Reshape  OutputDimensionality=Customize  OutputDimensions=[3,3]
  Singular Value Decomposition : dspfactors/Singular Value Decomposition  wantv=on  wanterr=off  SimulateUsing=Interpreted execution
  Terminator : Terminator
  Transpose1 : Math  Operator=transpose
  Vector Concatenate1 : Concatenate  NumInputs=3
  Abn_sens : Outport
  wires:
  Reshape1/1 -> Transpose1/1, Determinant of 3x3 Matrix1/1
  Reshape2/1 -> Determinant of 3x3 Matrix/1, Matrix Multiply2/1
  Vector Concatenate1/1 -> Create Diagonal Matrix1/1
  Transpose1/1 -> Matrix Multiply2/3
  Determinant of 3x3 Matrix1/1 -> Product1/2
  Product1/1 -> Vector Concatenate1/3
  Singular Value Decomposition/1 -> Reshape2/1
  Singular Value Decomposition/3 -> Reshape1/1
  Create Diagonal Matrix1/1 -> Matrix Multiply2/2
  Constant1/1 -> Vector Concatenate1/2, Vector Concatenate1/1
  Determinant of 3x3 Matrix/1 -> Product1/1
  B/1(Out1) -> Singular Value Decomposition/1
  Singular Value Decomposition/2 -> Terminator/1
  s1/1 -> B/1(s1)
  s2/1 -> B/2(s2)
  s3/1 -> B/3(s3)
  v1/1 -> B/4(v1)
  v2/1 -> B/5(v2)
  v3/1 -> B/6(v3)
  Matrix Multiply2/1 -> Abn_sens/1

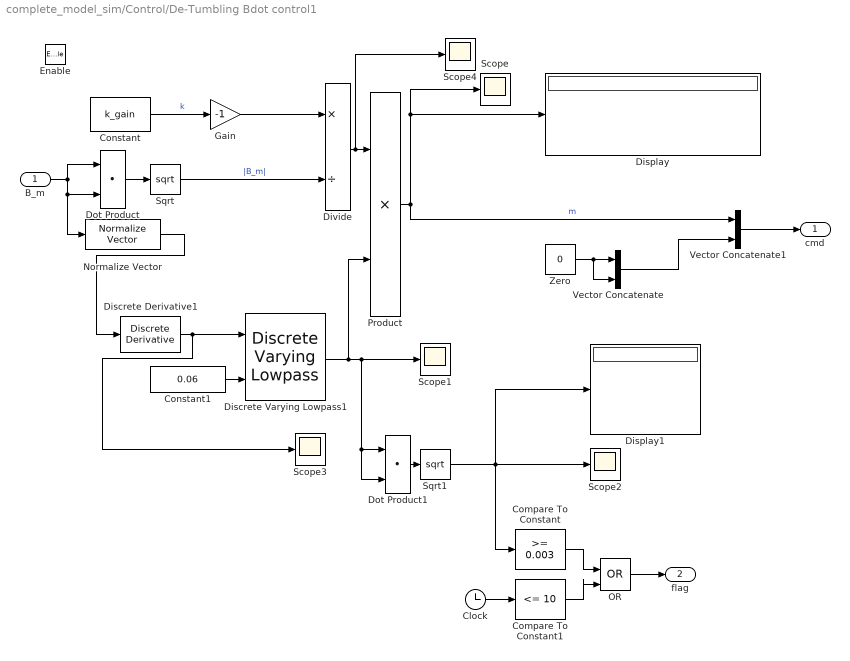
== system complete_model_sim/Control/De-Tumbling Bdot control1 ==
  B_m : Inport
  Enable : EnablePort
  Clock : Clock
  Compare To Constant : simulink/Logic and Bit Operations/Compare To Constant  relop=>=  const=0.003  OutDataTypeStr=boolean
  Compare To Constant1 : simulink/Logic and Bit Operations/Compare To Constant  relop=<=  const=10  OutDataTypeStr=boolean
  Constant : Constant  Value=k_gain
  Constant1 : Constant  Value=0.06  SampleTime=1/freq_mag
  Discrete Derivative1 : simulink/Discrete/Discrete Derivative  gainval=1.0  ICPrevScaledInput=0  OutMin=[]  OutMax=[]  OutDataType=fixdt(1, 16)  OutScaling=2^-10  DoSatur=off
  Discrete Varying Lowpass1 : cstblocks/Linear Parameter Varying/Discrete Varying Lowpass  N=1  w0=0  Ts=1/freq_mag
  Display : Display
  Display1 : Display
  Divide : Product  Inputs=*/
  Dot Product : DotProduct  OutDataTypeStr=Inherit: Inherit via internal rule
  Dot Product1 : DotProduct  OutDataTypeStr=Inherit: Inherit via internal rule
  Gain : Gain  Gain=-1
  Normalize Vector : vrlib/Utilities/Normalize Vector  maxzero=0
  OR : Logic  Operator=OR  IconShape=distinctive  AllPortsSameDT=off  OutDataTypeStr=boolean
  Product : Product
  Scope{,1..4} (5 alike) : Scope
  Sqrt : Sqrt
  Sqrt1 : Sqrt
  Vector Concatenate : Concatenate
  Vector Concatenate1 : Concatenate
  Zero : Constant  Value=0  OutDataTypeStr=Inherit: Inherit via back propagation
  cmd : Outport
  flag : Outport  Port=2
  wires:
  Dot Product/1 -> Sqrt/1
  Constant/1 -> Gain/1  "k"
  Divide/1 -> Scope4/1, Product/1
  Product/1 -> Vector Concatenate1/1, Scope/1, Display/1  "m"
  Sqrt/1 -> Divide/2  "|B_m|"
  Gain/1 -> Divide/1
  Normalize Vector/1 -> Discrete Derivative1/1
  B_m/1 -> Dot Product/2, Normalize Vector/1, Dot Product/1
  Discrete Derivative1/1 -> Discrete Varying Lowpass1/1, Scope3/1
  Sqrt1/1 -> Display1/1, Compare To Constant/1, Scope2/1
  Dot Product1/1 -> Sqrt1/1
  OR/1 -> flag/1
  Compare To Constant/1 -> OR/1
  Compare To Constant1/1 -> OR/2
  Clock/1 -> Compare To Constant1/1
  Constant1/1 -> Discrete Varying Lowpass1/2
  Discrete Varying Lowpass1/1 -> Scope1/1, Dot Product1/2, Dot Product1/1, Product/2
  Zero/1 -> Vector Concatenate/2, Vector Concatenate/1
  Vector Concatenate/1 -> Vector Concatenate1/2
  Vector Concatenate1/1 -> cmd/1

== system complete_model_sim/Control/Slew Maneuver ==
  Abn_sens : Inport
  Aln : Inport  Port=2
  B_m : Inport  Port=3
  Enable : EnablePort
  Control Logic : Subsystem
  Gain : Gain  Gain=-1
  Gain2 : Gain  Gain=-0.01
  Matrix Multiply : Product  Multiplication=Matrix(*)
  Scope : Scope
  Sum : Sum
  Transpose : Math  Operator=transpose
  compute alphadots : Subsystem
  compute alphas : Subsystem
  cmd : Outport
  wires:
  Aln/1 -> Transpose/1
  Transpose/1 -> Matrix Multiply/2
  Abn_sens/1 -> Matrix Multiply/1, compute alphadots/1(Abn)
  Matrix Multiply/1 -> compute alphas/1(Abl), compute alphadots/2(Abl)
  compute alphadots/1(Alphadots) -> Gain/1
  compute alphas/1(estimated state) -> Scope/1, Gain2/1
  Gain/1 -> Sum/1
  Gain2/1 -> Sum/2
  B_m/1 -> Control Logic/2(B_m)
  Sum/1 -> Control Logic/1(u)
  Control Logic/1(cmd) -> cmd/1

== system complete_model_sim/Control Logic/Subsystem ==
  Bm : Inport
  u : Inport  Port=2
  Enable : EnablePort
  Assembly Matrix : Subsystem
  Constant : Constant  Value=0
  Constant1 : Constant  Value=0
  LU Solver : dspsolvers/LU Solver
  Selector : Selector  InputPortWidth=3  IndexOptions=Index vector (dialog)  Indices=1  OutputSizes=1
  Selector1 : Selector  InputPortWidth=3  IndexOptions=Index vector (dialog)  Indices=3  OutputSizes=1
  Selector2 : Selector  InputPortWidth=3  IndexOptions=Index vector (dialog)  Indices=2  OutputSizes=1
  Vector Concatenate : Concatenate  NumInputs=5
  Out1 : Outport
  wires:
  Bm/1 -> Assembly Matrix/1(Bm)
  Assembly Matrix/1(Matrix) -> LU Solver/1
  u/1 -> LU Solver/2
  LU Solver/1 -> Selector2/1, Selector1/1, Selector/1
  Selector/1 -> Vector Concatenate/1
  Constant/1 -> Vector Concatenate/2
  Selector1/1 -> Vector Concatenate/3
  Constant1/1 -> Vector Concatenate/4
  Selector2/1 -> Vector Concatenate/5
  Vector Concatenate/1 -> Out1/1

== system complete_model_sim/Control Logic/Subsystem1 ==
  B_m : Inport
  u : Inport  Port=2
  Enable : EnablePort
  Assembly Matrix : Subsystem
  Constant : Constant  Value=0
  Constant1 : Constant  Value=0
  LU Solver : dspsolvers/LU Solver
  Selector : Selector  InputPortWidth=3  IndexOptions=Index vector (dialog)  Indices=2  OutputSizes=1
  Selector1 : Selector  InputPortWidth=3  IndexOptions=Index vector (dialog)  Indices=3  OutputSizes=1
  Selector2 : Selector  InputPortWidth=3  IndexOptions=Index vector (dialog)  Indices=1  OutputSizes=1
  Vector Concatenate : Concatenate  NumInputs=5
  Out1 : Outport
  wires:
  Assembly Matrix/1("Matrix ") -> LU Solver/1
  B_m/1 -> Assembly Matrix/1(B_m)
  u/1 -> LU Solver/2
  Selector1/1 -> Vector Concatenate/3
  Selector/1 -> Vector Concatenate/2
  Constant/1 -> Vector Concatenate/1
  Selector2/1 -> Vector Concatenate/4
  Constant1/1 -> Vector Concatenate/5
  LU Solver/1 -> Selector2/1, Selector1/1, Selector/1
  Vector Concatenate/1 -> Out1/1

== system complete_model_sim/Control Logic/norm ==
  In1 : Inport
  Dot Product : DotProduct  OutDataTypeStr=Inherit: Inherit via internal rule
  Sqrt : Sqrt
  Out1 : Outport
  wires:
  In1/1 -> Dot Product/1, Dot Product/2
  Dot Product/1 -> Sqrt/1
  Sqrt/1 -> Out1/1

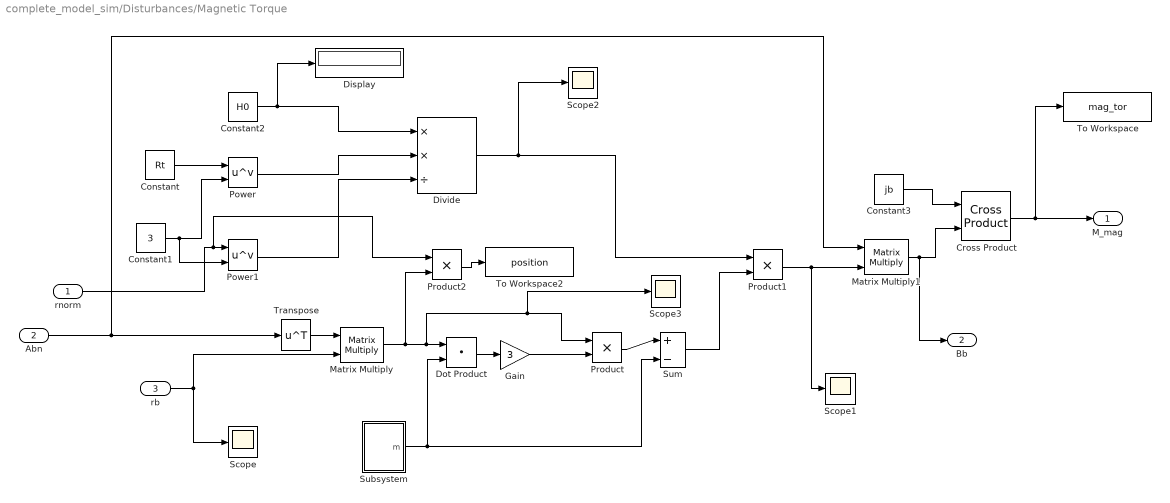
== system complete_model_sim/Disturbances/Magnetic Torque  ==
  rnorm : Inport
  Abn : Inport  Port=2
  rb : Inport  Port=3
  Constant : Constant  Value=Rt
  Constant1 : Constant  Value=3
  Constant2 : Constant  Value=H0
  Constant3 : Constant  Value=jb
  Cross Product : matrix_library/Cross Product
  Display : Display
  Divide : Product  Inputs=**/
  Dot Product : DotProduct  OutDataTypeStr=Inherit: Inherit via internal rule
  Gain : Gain  Gain=3
  Matrix Multiply : Product  Multiplication=Matrix(*)
  Matrix Multiply1 : Product  Multiplication=Matrix(*)
  Power : Math  Operator=pow
  Power1 : Math  Operator=pow
  Product : Product
  Product1 : Product
  Product2 : Product
  Scope{,1..3} (4 alike) : Scope
  Subsystem : Subsystem
  Sum : Sum  Inputs=|+-
  To Workspace : ToWorkspace  VariableName=mag_tor  SampleTime=-1
  To Workspace2 : ToWorkspace  VariableName=position  SampleTime=-1
  Transpose : Math  Operator=transpose
  M_mag : Outport
  Bb : Outport  Port=2
  wires:
  Abn/1 -> Matrix Multiply1/1, Transpose/1
  Transpose/1 -> Matrix Multiply/1
  rb/1 -> Scope/1, Matrix Multiply/2
  Matrix Multiply/1 -> Product2/2, Scope3/1, Product/1, Dot Product/1
  Subsystem/1(m) -> Sum/2, Dot Product/2
  Dot Product/1 -> Gain/1
  Gain/1 -> Product/2
  Product/1 -> Sum/1
  Constant/1 -> Power/1
  Constant1/1 -> Power1/2, Power/2
  rnorm/1 -> Product2/1, Power1/1
  Constant2/1 -> Display/1, Divide/1
  Power/1 -> Divide/2
  Power1/1 -> Divide/3
  Divide/1 -> Scope2/1, Product1/1
  Sum/1 -> Product1/2
  Product1/1 -> Scope1/1, Matrix Multiply1/2
  Constant3/1 -> Cross Product/1
  Matrix Multiply1/1 -> Bb/1, Cross Product/2
  Cross Product/1 -> To Workspace/1, M_mag/1
  Product2/1 -> To Workspace2/1

== system complete_model_sim/Disturbances/gravity torque ==
  c : Inport
  Input : Inport  Port=2
  Constant : Constant  Value=mu
  Constant1 : Constant  Value=I
  Constant3 : Constant  Value=3
  Cross Product : matrix_library/Cross Product
  Divide : Product  Inputs=**/
  Gain : Gain  Gain=-1
  Matrix Multiply : Product  Multiplication=Matrix(*)
  Power : Math  Operator=pow
  Product : Product
  Mg : Outport
  wires:
  Constant1/1 -> Matrix Multiply/1
  c/1 -> Matrix Multiply/2, Cross Product/2
  Matrix Multiply/1 -> Cross Product/1
  Constant3/1 -> Power/2, Divide/2
  Power/1 -> Divide/3
  Constant/1 -> Divide/1
  Divide/1 -> Gain/1
  Gain/1 -> Product/2
  Cross Product/1 -> Product/1
  Product/1 -> Mg/1
  Input/1 -> Power/1

== system complete_model_sim/Horizon Sensor/EH sensor modeling ==
  rb : Inport
  Cross Product : matrix_library/Cross Product
  Normalize Vector : vrlib/Utilities/Normalize Vector  maxzero=0
  Product : Product
  Sum2 : Sum
  Uniform Random Number : UniformRandomNumber  SampleTime=1/30
  Uniform Random Number1 : UniformRandomNumber  SampleTime=1/30
  Uniform Random Number2 : UniformRandomNumber  SampleTime=1/30
  Uniform Random Number3 : UniformRandomNumber  Minimum=0  Maximum=tan(deg2rad(0.1))*0.1  SampleTime=1/30
  Vector Concatenate : Concatenate  NumInputs=3
  Zero-Order Hold : ZeroOrderHold  SampleTime=1/freq_earth
  q : Outport
  wires:
  Product/1 -> Sum2/1
  Uniform Random Number3/1 -> Product/1
  Uniform Random Number1/1 -> Vector Concatenate/2
  Uniform Random Number2/1 -> Vector Concatenate/3
  Normalize Vector/1 -> Product/2
  Uniform Random Number/1 -> Vector Concatenate/1
  Zero-Order Hold/1 -> Cross Product/2, Sum2/2  "R_B"
  Vector Concatenate/1 -> Cross Product/1
  Cross Product/1 -> Normalize Vector/1
  Sum2/1 -> q/1  "q"
  rb/1 -> Zero-Order Hold/1

== system complete_model_sim/Horizon Sensor/FOV CHECK ==
  rb : Inport
  Acos : Trigonometry  Operator=acos
  Dot Product : DotProduct  OutDataTypeStr=Inherit: Inherit via internal rule
  FOV angle : Constant  Value=FOV_earth
  Gain : Gain  Gain=-1
  Less Than : RelationalOperator  Operator=<  OutDataTypeStr=boolean  RndMeth=Simplest  InputSameDT=off
  optical axis : Constant  Value=[-1;0;0]
  b : Outport
  wires:
  optical axis/1 -> Dot Product/1
  Dot Product/1 -> Acos/1
  FOV angle/1 -> Less Than/2
  Acos/1 -> Less Than/1
  Less Than/1 -> b/1
  Gain/1 -> Dot Product/2
  rb/1 -> Gain/1

== system complete_model_sim/Kinematics/Kinematics 312 ==
  w : Inport
  Enable : EnablePort  StatesWhenEnabling=reset
  A - s_312 : Subsystem
  Euler angles : Subsystem
  IC : InitialCondition  Value=s0
  s_312 - A : Subsystem
  s_313 - A : Subsystem
  A : Outport
  wires:
  s_312 - A/1(A) -> A/1  "A"
  Euler angles/1(s) -> s_312 - A/1(s)  "s"
  w/1 -> Euler angles/1(w)
  IC/1 -> Euler angles/2(s0)
  A - s_312/1(s) -> IC/1
  s_313 - A/1(A) -> A - s_312/1(A)
  [s_313] -> s_313 - A/1(s)

== system complete_model_sim/Kinematics/Kinematics 313 ==
  w : Inport
  Enable : EnablePort  StatesWhenEnabling=reset
  A - s_313 : Subsystem
  Euler angles : Subsystem
  s_312 - A : Subsystem
  s_313 - A : Subsystem
  A : Outport
  wires:
  w/1 -> Euler angles/1(w)
  Euler angles/1(s) -> s_313 - A/1(s)
  s_313 - A/1(A) -> A/1
  A - s_313/1(s) -> Euler angles/2(s0)
  s_312 - A/1(A) -> A - s_313/1(A)
  [s_312] -> s_312 - A/1(s)

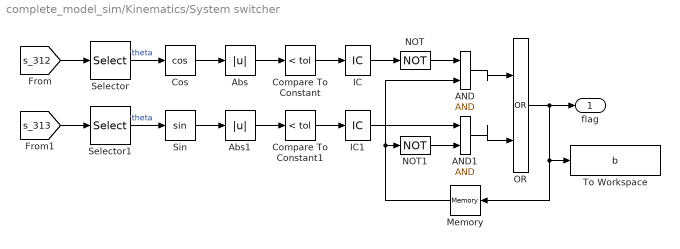
== system complete_model_sim/Kinematics/System switcher ==
  AND : Logic  IconShape=distinctive  AllPortsSameDT=off  OutDataTypeStr=boolean
  AND1 : Logic  IconShape=distinctive  AllPortsSameDT=off  OutDataTypeStr=boolean
  Abs : Abs  SaturateOnIntegerOverflow=off
  Abs1 : Abs  SaturateOnIntegerOverflow=off
  Compare To Constant : simulink/Logic and Bit Operations/Compare To Constant  relop=<  const=tol  OutDataTypeStr=boolean
  Compare To Constant1 : simulink/Logic and Bit Operations/Compare To Constant  relop=<  const=tol  OutDataTypeStr=boolean
  Cos : Trigonometry  Operator=cos
  IC : InitialCondition  Value=0
  IC1 : InitialCondition  Value=0
  Memory : Memory  InitialCondition=1
  NOT : Logic  Operator=NOT  IconShape=distinctive  AllPortsSameDT=off  OutDataTypeStr=boolean
  NOT1 : Logic  Operator=NOT  IconShape=distinctive  AllPortsSameDT=off  OutDataTypeStr=boolean
  OR : Logic  Operator=OR  IconShape=distinctive  AllPortsSameDT=off  OutDataTypeStr=boolean
  Selector : Selector  InputPortWidth=3  IndexOptions=Index vector (dialog)  Indices=2  OutputSizes=1
  Selector1 : Selector  InputPortWidth=3  IndexOptions=Index vector (dialog)  Indices=2  OutputSizes=1
  Sin : Trigonometry
  To Workspace : ToWorkspace  VariableName=b  SaveFormat=Timeseries  SampleTime=-1
  flag : Outport
  wires:
  Cos/1 -> Abs/1
  [s_312] -> Selector/1
  Compare To Constant/1 -> IC/1
  Selector1/1 -> Sin/1  "theta"
  Abs/1 -> Compare To Constant/1
  Compare To Constant1/1 -> IC1/1
  Selector/1 -> Cos/1  "theta"
  Abs1/1 -> Compare To Constant1/1
  Sin/1 -> Abs1/1
  [s_313] -> Selector1/1
  IC/1 -> NOT/1
  NOT/1 -> AND/1
  AND/1 -> OR/1
  NOT1/1 -> AND1/2
  IC1/1 -> AND1/1
  AND1/1 -> OR/2
  OR/1 -> To Workspace/1, Memory/1, flag/1
  Memory/1 -> AND/2, NOT1/1

== system complete_model_sim/Slew Maneuver/compute alphadots ==
  Abn : Inport
  Abl : Inport  Port=2
  Constant : Constant
  Constant1 : Constant  Value=[0;0;n]
  Discrete Derivative : simulink/Discrete/Discrete Derivative  gainval=1.0  ICPrevScaledInput=0.0  OutMin=[]  OutMax=[]  OutDataType=fixdt(1, 16)  OutScaling=2^-10  DoSatur=off
  Discrete Varying Lowpass : cstblocks/Linear Parameter Varying/Discrete Varying Lowpass  N=1  w0=0  Ts=1/30
  Gain : Gain  Gain=-1
  Invert 3x3 Matrix : aerolibutil/Invert  3x3 Matrix
  Matrix Multiply1 : Product  Multiplication=Matrix(*)
  Matrix Multiply2 : Product  Multiplication=Matrix(*)
  Scope3 : Scope
  Selector : Selector  NumberOfDimensions=2  InputPortWidth=3  IndexOptions=Index vector (dialog),Index vector (dialog)  Indices=3,2  OutputSizes=1,1
  Selector1 : Selector  NumberOfDimensions=2  InputPortWidth=3  IndexOptions=Index vector (dialog),Index vector (dialog)  Indices=1,3  OutputSizes=1,1
  Selector2 : Selector  NumberOfDimensions=2  InputPortWidth=3  IndexOptions=Index vector (dialog),Index vector (dialog)  Indices=2,1  OutputSizes=1,1
  Sum : Sum  Inputs=-+
  Vector Concatenate : Concatenate  NumInputs=3
  Alphadots : Outport
  wires:
  Selector/1 -> Vector Concatenate/1
  Matrix Multiply2/1 -> Sum/1
  Discrete Varying Lowpass/1 -> Matrix Multiply1/1
  Matrix Multiply1/1 -> Gain/1
  Constant1/1 -> Matrix Multiply2/2
  Abn/1 -> Invert 3x3 Matrix/1, Discrete Derivative/1
  Invert 3x3 Matrix/1 -> Matrix Multiply1/2
  Gain/1 -> Selector2/1, Selector1/1, Selector/1
  Constant/1 -> Discrete Varying Lowpass/2
  Sum/1 -> Alphadots/1
  Selector2/1 -> Vector Concatenate/3
  Selector1/1 -> Vector Concatenate/2
  Discrete Derivative/1 -> Discrete Varying Lowpass/1
  Vector Concatenate/1 -> Sum/2, Scope3/1
  Abl/1 -> Matrix Multiply2/1

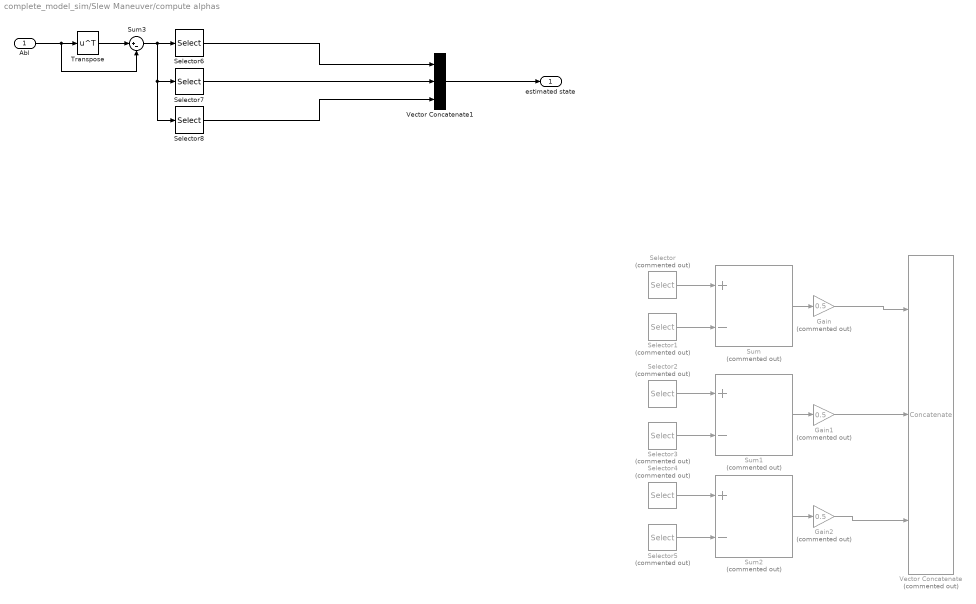
== system complete_model_sim/Slew Maneuver/compute alphas ==
  Abl : Inport
  Gain : Gain  Commented=on  Gain=0.5
  Gain1 : Gain  Commented=on  Gain=0.5
  Gain2 : Gain  Commented=on  Gain=0.5
  Selector : Selector  Commented=on  NumberOfDimensions=2  InputPortWidth=3  IndexOptions=Index vector (dialog),Index vector (dialog)  Indices=2,3  OutputSizes=1,1
  Selector1 : Selector  Commented=on  NumberOfDimensions=2  InputPortWidth=3  IndexOptions=Index vector (dialog),Index vector (dialog)  Indices=3,2  OutputSizes=1,1
  Selector2 : Selector  Commented=on  NumberOfDimensions=2  InputPortWidth=3  IndexOptions=Index vector (dialog),Index vector (dialog)  Indices=3,1  OutputSizes=1,1
  Selector3 : Selector  Commented=on  NumberOfDimensions=2  InputPortWidth=3  IndexOptions=Index vector (dialog),Index vector (dialog)  Indices=1,3  OutputSizes=1,1
  Selector4 : Selector  Commented=on  NumberOfDimensions=2  InputPortWidth=3  IndexOptions=Index vector (dialog),Index vector (dialog)  Indices=1,2  OutputSizes=1,1
  Selector5 : Selector  Commented=on  NumberOfDimensions=2  InputPortWidth=3  IndexOptions=Index vector (dialog),Index vector (dialog)  Indices=2,1  OutputSizes=1,1
  Selector6 : Selector  NumberOfDimensions=2  InputPortWidth=3  IndexOptions=Index vector (dialog),Index vector (dialog)  Indices=3,2  OutputSizes=1,1
  Selector7 : Selector  NumberOfDimensions=2  InputPortWidth=3  IndexOptions=Index vector (dialog),Index vector (dialog)  Indices=1,3  OutputSizes=1,1
  Selector8 : Selector  NumberOfDimensions=2  InputPortWidth=3  IndexOptions=Index vector (dialog),Index vector (dialog)  Indices=2,1  OutputSizes=1,1
  Sum : Sum  Commented=on  Inputs=+-
  Sum1 : Sum  Commented=on  Inputs=+-
  Sum2 : Sum  Commented=on  Inputs=+-
  Sum3 : Sum  Inputs=|+-
  Transpose : Math  Operator=transpose
  Vector Concatenate : Concatenate  Commented=on  NumInputs=3
  Vector Concatenate1 : Concatenate  NumInputs=3
  estimated state : Outport
  wires:
  Selector1/1 -> Sum/2
  Selector/1 -> Sum/1
  Sum/1 -> Gain/1
  Selector2/1 -> Sum1/1
  Selector3/1 -> Sum1/2
  Selector4/1 -> Sum2/1
  Selector5/1 -> Sum2/2
  Sum1/1 -> Gain1/1
  Sum2/1 -> Gain2/1
  Gain/1 -> Vector Concatenate/1
  Gain1/1 -> Vector Concatenate/2
  Gain2/1 -> Vector Concatenate/3
  Abl/1 -> Sum3/2, Transpose/1
  Transpose/1 -> Sum3/1
  Sum3/1 -> Selector8/1, Selector7/1, Selector6/1
  Vector Concatenate1/1 -> estimated state/1
  Selector7/1 -> Vector Concatenate1/2
  Selector6/1 -> Vector Concatenate1/1
  Selector8/1 -> Vector Concatenate1/3

== system complete_model_sim/Sun Sensor/FOV CHECK ==
  In1 : Inport
  Acos : Trigonometry  Operator=acos
  Dot Product : DotProduct  OutDataTypeStr=Inherit: Inherit via internal rule
  FOV angle : Constant  Value=FOV_sun
  Less Than : RelationalOperator  Operator=<  OutDataTypeStr=boolean  RndMeth=Simplest  InputSameDT=off
  optical axis : Constant  Value=[0;0;1]
  b : Outport
  wires:
  optical axis/1 -> Dot Product/1
  In1/1 -> Dot Product/2
  Dot Product/1 -> Acos/1
  FOV angle/1 -> Less Than/2
  Acos/1 -> Less Than/1
  Less Than/1 -> b/1

== system complete_model_sim/Sun Sensor/Sun Sensor Modeling ==
  Sb : Inport
  Cross Product : matrix_library/Cross Product
  Normalize Vector : vrlib/Utilities/Normalize Vector  maxzero=0
  Normalize Vector1 : vrlib/Utilities/Normalize Vector  maxzero=0
  Product : Product
  Random Number : RandomNumber  Variance=tan(deg2rad(1/60))^2*0.1  SampleTime=0.1
  Sum2 : Sum
  Uniform Random Number : UniformRandomNumber  SampleTime=1/freq_sun
  Uniform Random Number1 : UniformRandomNumber  SampleTime=1/freq_sun
  Uniform Random Number2 : UniformRandomNumber  SampleTime=1/freq_sun
  Vector Concatenate : Concatenate  NumInputs=3
  Zero-Order Hold : ZeroOrderHold  SampleTime=1/freq_sun
  s3 : Outport
  wires:
  Zero-Order Hold/1 -> Cross Product/2, Sum2/2  "Sb"
  Sum2/1 -> Normalize Vector/1  "q"
  Uniform Random Number1/1 -> Vector Concatenate/2
  Vector Concatenate/1 -> Cross Product/1
  Uniform Random Number2/1 -> Vector Concatenate/3
  Normalize Vector/1 -> s3/1
  Uniform Random Number/1 -> Vector Concatenate/1
  Product/1 -> Sum2/1
  Random Number/1 -> Product/1
  Sb/1 -> Zero-Order Hold/1
  Cross Product/1 -> Normalize Vector1/1
  Normalize Vector1/1 -> Product/2

== system complete_model_sim/kep_dyn/r_norm ==
  e : Inport
  theta : Inport  Port=2
  Constant : Constant  Value=a
  Constant1 : Constant
  Cos : Trigonometry  Operator=cos
  Divide : Product  Inputs=*/
  Power : Math  Operator=magnitude^2
  Product : Product
  Product1 : Product
  Sum : Sum  Inputs=+-
  Sum2 : Sum
  r : Outport
  wires:
  e/1 -> Product1/2, Power/1
  Power/1 -> Sum/2
  Constant1/1 -> Sum2/2, Sum/1
  Sum/1 -> Product/2
  Constant/1 -> Product/1
  theta/1 -> Cos/1
  Cos/1 -> Product1/1
  Product1/1 -> Sum2/1
  Product/1 -> Divide/1
  Sum2/1 -> Divide/2
  Divide/1 -> r/1

== system complete_model_sim/kep_dyn/theta integration ==
  theta : Inport
  e : Inport  Port=2
  Constant : Constant  Value=n
  Constant2 : Constant
  Constant3 : Constant  Value=3/2
  Cos : Trigonometry  Operator=cos
  Divide : Product  Inputs=*/
  Math Function : Math  Operator=square
  Math Function1 : Math  Operator=square
  Math Function2 : Math  Operator=pow
  Product : Product
  Product1 : Product
  Sum : Sum
  Sum1 : Sum  Inputs=+-
  theta_dot : Outport
  wires:
  Product1/1 -> Divide/1
  Product/1 -> Sum/2
  Math Function2/1 -> Divide/2
  Sum1/1 -> Math Function2/1
  Constant2/1 -> Sum1/1, Sum/1
  Math Function1/1 -> Sum1/2
  e/1 -> Product/2, Math Function1/1
  Constant3/1 -> Math Function2/2
  Constant/1 -> Product1/1
  Sum/1 -> Math Function/1
  Math Function/1 -> Product1/2
  Cos/1 -> Product/1
  theta/1 -> Cos/1
  Divide/1 -> theta_dot/1

== system complete_model_sim/relative kinematics/Subsystem ==
  theta : Inport
  Constant3 : Constant
  Constant4 : Constant  Value=0
  Cos2 : Trigonometry  Operator=cos
  Cos3 : Trigonometry
  Gain : Gain  Gain=-1
  Matrix Concatenate1 : Concatenate  NumInputs=3  Mode=Multidimensional array  ConcatenateDimension=2
  Vector Concatenate : Concatenate  NumInputs=3
  Vector Concatenate1 : Concatenate  NumInputs=3
  Vector Concatenate2 : Concatenate  NumInputs=3
  A_PL : Outport
  wires:
  Constant4/1 -> Vector Concatenate2/2, Vector Concatenate/3, Vector Concatenate1/3, Vector Concatenate2/1
  Vector Concatenate/1 -> Matrix Concatenate1/1
  Cos2/1 -> Vector Concatenate1/2, Vector Concatenate/1
  Gain/1 -> Vector Concatenate1/1
  Cos3/1 -> Vector Concatenate/2, Gain/1
  Constant3/1 -> Vector Concatenate2/3
  Vector Concatenate2/1 -> Matrix Concatenate1/3
  Vector Concatenate1/1 -> Matrix Concatenate1/2
  theta/1 -> Cos2/1, Cos3/1
  Matrix Concatenate1/1 -> A_PL/1  "A_PL"

== system complete_model_sim/Attitude Determination  1/Enabled Subsystem/S ==
  q : Inport
  p : Inport  Port=2
  Cross Product : matrix_library/Cross Product
  Cross Product1 : matrix_library/Cross Product
  Matrix Concatenate : Concatenate  NumInputs=3  Mode=Multidimensional array  ConcatenateDimension=2
  Normalize Vector : vrlib/Utilities/Normalize Vector  maxzero=0
  S : Outport
  wires:
  p/1 -> Matrix Concatenate/1, Cross Product/1, Cross Product1/1
  q/1 -> Cross Product/2
  Normalize Vector/1 -> Matrix Concatenate/2, Cross Product1/2
  Matrix Concatenate/1 -> S/1
  Cross Product1/1 -> Matrix Concatenate/3
  Cross Product/1 -> Normalize Vector/1

== system complete_model_sim/Attitude Determination  1/Enabled Subsystem/V ==
  b : Inport
  a : Inport  Port=2
  Cross Product : matrix_library/Cross Product
  Cross Product1 : matrix_library/Cross Product
  Matrix Concatenate : Concatenate  NumInputs=3  Mode=Multidimensional array  ConcatenateDimension=2
  Normalize Vector : vrlib/Utilities/Normalize Vector  maxzero=0
  V : Outport
  wires:
  Cross Product1/1 -> Matrix Concatenate/3
  Matrix Concatenate/1 -> V/1
  Normalize Vector/1 -> Cross Product1/2, Matrix Concatenate/2
  Cross Product/1 -> Normalize Vector/1
  b/1 -> Cross Product/2
  a/1 -> Cross Product1/1, Cross Product/1, Matrix Concatenate/1

== system complete_model_sim/Attitude Determination  1/Statistical Method/B ==
  s1 : Inport
  s2 : Inport  Port=2
  s3 : Inport  Port=3
  v1 : Inport  Port=4
  v2 : Inport  Port=5
  v3 : Inport  Port=6
  Gain : Gain  Gain=alpha1
  Gain1 : Gain  Gain=alpha2
  Gain2 : Gain  Gain=alpha3
  Matrix Multiply : Product  Multiplication=Matrix(*)
  Matrix Multiply1 : Product  Multiplication=Matrix(*)
  Matrix Multiply2 : Product  Multiplication=Matrix(*)
  Sum : Sum  Inputs=+++
  Transpose : Math  Operator=transpose
  Transpose1 : Math  Operator=transpose
  Transpose2 : Math  Operator=transpose
  Out1 : Outport
  wires:
  v1/1 -> Transpose/1
  Transpose/1 -> Matrix Multiply/2
  s1/1 -> Matrix Multiply/1
  Transpose1/1 -> Matrix Multiply1/2
  s2/1 -> Matrix Multiply1/1
  Transpose2/1 -> Matrix Multiply2/2
  v3/1 -> Transpose2/1
  Sum/1 -> Out1/1
  Matrix Multiply/1 -> Gain/1
  Matrix Multiply1/1 -> Gain1/1
  Matrix Multiply2/1 -> Gain2/1
  Gain/1 -> Sum/1
  Gain1/1 -> Sum/2
  Gain2/1 -> Sum/3
  v2/1 -> Transpose1/1
  s3/1 -> Matrix Multiply2/1
